simulink model "relay"  (R2015a)
settings: Solver=ode45  StartTime=0.0  StopTime=160  RelTol=1e-3
settings Model: Creator=ra428  LastModifiedBy=ra428

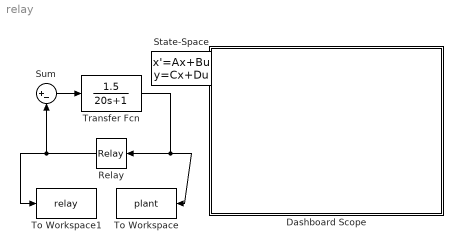
== system relay ==
  Dashboard Scope : Subsystem  DialogController=hmiCreateDDGDialog  IsWebBlock=on  mask(MathWorksWebBlock){webBlockId=21035071-f40a-4a66-bff0-c6b7fbc0910f, webBlockType=sdiscope, ShowInitialText=on, HMISrcModelName=untitled}
      mask prompts: webBlockId "WebBlock Id"; webBlockType "WebBlock Type"; HMISrcModelName "Source Model"
      mask Help: helpview([docroot '/mapfiles/simulink.map'], 'hmi_scope')
      mask Display:
      | if strcmp(get_param(bdroot(gcb),'BlockDiagramType'), 'library')
      |     image([(matlabroot) '/toolbox/simulink/hmi/icons/DashboardScope.png']);
      | end
  Relay : Relay  OnSwitchValue=1  OffSwitchValue=-1  OnOutputValue=1.5  OffOutputValue=-1
  State-Space : StateSpace  A=[-1 1 0; 0 -1 1; 0 0 -1]  B=[0;0;1]  C=[1.5 0 0 ]  D=0  X0=0
  Sum : Sum  Inputs=|+-
  To Workspace : ToWorkspace  VariableName=plant  SaveFormat=Timeseries  SampleTime=-1
  To Workspace1 : ToWorkspace  VariableName=relay  SaveFormat=Timeseries  SampleTime=-1
  Transfer Fcn : TransferFcn  Numerator=[1.5]  Denominator=[20 1]
  wires:
  Transfer Fcn/1 -> To Workspace/1, Relay/1
  Relay/1 -> Sum/2, To Workspace1/1
  Sum/1 -> Transfer Fcn/1

== system relay/Dashboard Scope ==
